simulink model "testing"  (R2023a)
settings: Solver=VariableStepAuto  StartTime=0.0  StopTime=200  RelTol=1e-3
model workspace (MAT data in the model file):
  K = Simulink.Parameter
  K.Value = 1
  K.DataType = 'auto'
  K.Complexity = 'real'
  K.Dimensions = [1 1]
  r = Simulink.Parameter
  r.Value = 1
  r.DataType = 'auto'
  r.Complexity = 'real'
  r.Dimensions = [1 1]
libraries: simulink x1
settings Model: Creator=Lucca  LastModifiedBy=Lucca

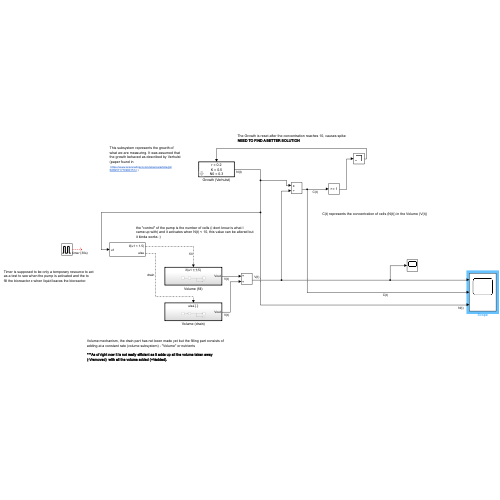
[thumbnail: Simulink's stored preview of the top-level diagram]
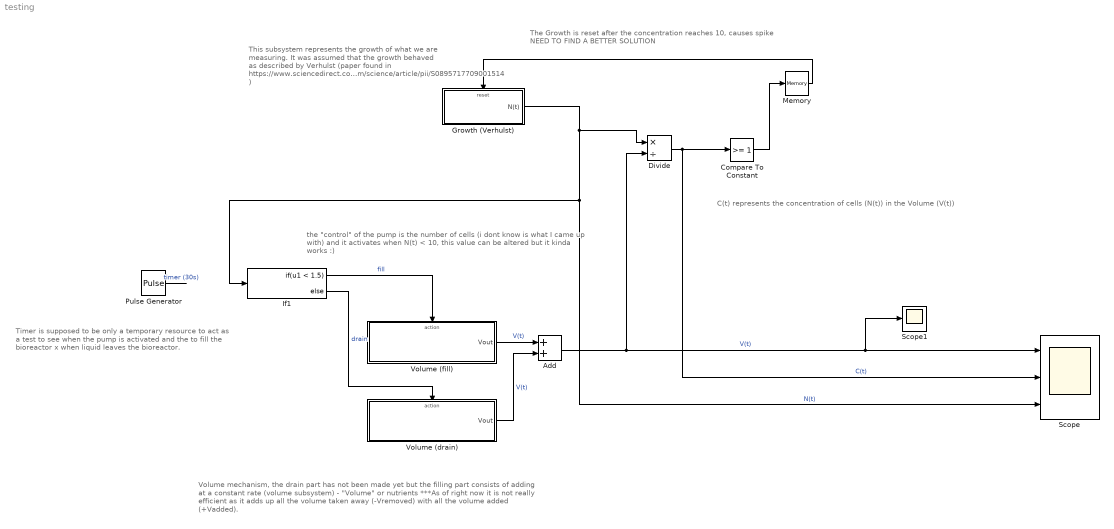
== system testing ==
  note: The Growth is reset after the concentration reaches 10, causes spike
      | NEED TO FIND A BETTER SOLUTION
  note: the "control" of the pump is the number of cells (i dont know is what I
      | came up with) and it activates when N(t) < 10, this value can be altered but
      | it kinda works :)
  note: Timer is supposed to be only a temporary resource to act
      | as a test to see when the pump is activated and the to
      | fill the bioreactor x when liquid leaves the bioreactor.
  note: C(t) represents the concentration of cells (N(t)) in the Volume (V(t))
  note: Volume mechanism, the drain part has not been made yet but the filling part consists of adding at a constant rate (volume subsystem) - "Volume" or nutrients
      |
      | ***As of right now it is not really efficient as it adds up all the volume taken away
      | (-Vremoved) with all the volume added (+Vadded).
  note: This subsystem represents the growth of
      | what we are measuring. It was assumed that
      | the growth behaved as described by Verhulst
      | (paper found in
      | https://www.sciencedirect.com/science/article/pii/S0895717709001514 )
  Add : Sum
  Compare To Constant : simulink/Logic and Bit Operations/Compare To Constant  relop=>=  const=1  OutDataTypeStr=boolean
  Divide : Product  Inputs=*/
  Growth (Verhulst) : Subsystem  mask{r=0.2, K=0.5, Ni=0.3}
      mask prompts: r "r - growth rate"; K "K - equilibrium value"; Ni "Ni - initial conditions"
      mask init:
      | str1 = "r = " + r;
      | str2 = "K = " + K;
      | str3 = "N0 = " + Ni;
      | label = [str1; str2; str3];
      mask Display: disp(label);
  If1 : If  IfExpression=u1 < 1.5
  Memory : Memory
  Pulse Generator : DiscretePulseGenerator  PulseType=Time based  Period=30  PulseWidth=50
  Scope : Scope  NumInputPorts=3
  Scope1 : Scope
  Volume (drain) : Subsystem
  Volume (fill) : Subsystem
  wires:
  Growth (Verhulst)/1(N(t)) -> If1/1, Scope/3, Divide/1  "N(t)"
  Compare To Constant/1 -> Memory/1
  Divide/1 -> Scope/2, Compare To Constant/1  "C(t)"
  Memory/1 -> Growth (Verhulst)/Reset
  Pulse Generator/1 -> ?  "timer (30s)"
  If1/1 -> Volume (fill)/Action  "fill"
  Add/1 -> Divide/2, Scope/1, Scope1/1  "V(t)"
  If1/2 -> Volume (drain)/Action  "drain"
  Volume (fill)/1(Vout) -> Add/1  "V(t)"
  Volume (drain)/1(Vout) -> Add/2  "V(t)"

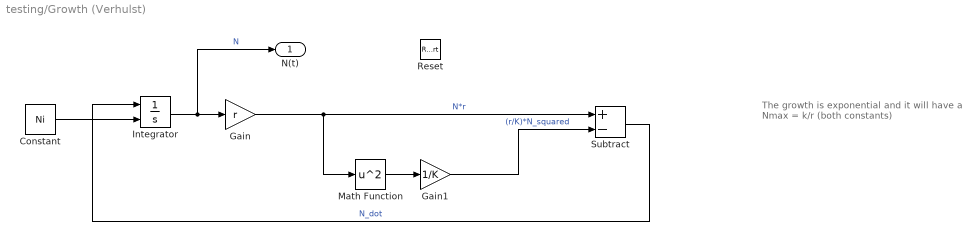
== system testing/Growth (Verhulst) ==
  note: The growth is exponential and it will have a
      | Nmax = k/r (both constants)
  Reset : ResetPort  DisableCoverage=on
  Constant : Constant  Value=Ni
  Gain : Gain  Gain=r
  Gain1 : Gain  Gain=1/K
  Integrator : Integrator  InitialConditionSource=external  InitialCondition=Ni
  Math Function : Math  Operator=square
  Subtract : Sum  Inputs=+-
  N(t) : Outport
  wires:
  Subtract/1 -> Integrator/1  "N_dot"
  Math Function/1 -> Gain1/1
  Gain/1 -> Subtract/1, Math Function/1  "N*r"
  Gain1/1 -> Subtract/2  "(r/K)*N_squared"
  Integrator/1 -> N(t)/1, Gain/1  "N"
  Constant/1 -> Integrator/2

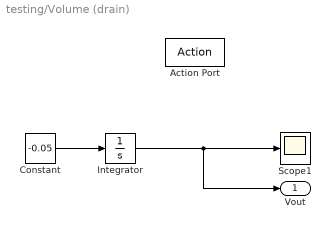
== system testing/Volume (drain) ==
  Action Port : ActionPort  ActionPortLabel=else
  Constant : Constant  Value=-0.05
  Integrator : Integrator  InitialCondition=0.2
  Scope1 : Scope
  Vout : Outport
  wires:
  Integrator/1 -> Scope1/1, Vout/1
  Constant/1 -> Integrator/1

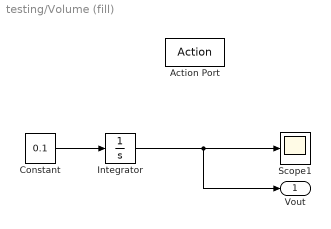
== system testing/Volume (fill) ==
  Action Port : ActionPort  ActionPortLabel=if(u1 < 1.5)
  Constant : Constant  Value=0.1
  Integrator : Integrator  InitialCondition=0.5
  Scope1 : Scope
  Vout : Outport
  wires:
  Integrator/1 -> Scope1/1, Vout/1
  Constant/1 -> Integrator/1
